simulink model "test6_1"  (R2014a)
settings: Solver=ode45  StartTime=0.0  StopTime=10.0  RelTol=1e-3
libraries: commrandsrc2 x1, commnoisgen2 x1
settings Model: Creator=asus  LastModifiedBy=asus

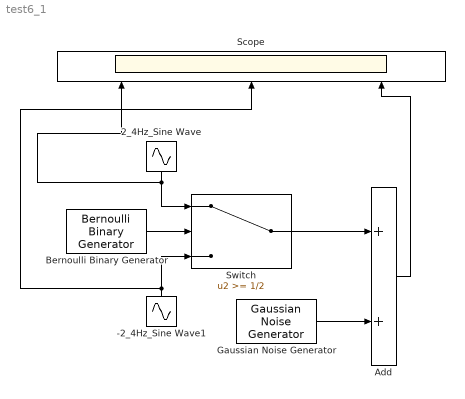
== system test6_1 ==
  -2_4Hz_Sine Wave1 : Sin  Amplitude=-2  Frequency=pi  SampleTime=1/8000
  2_4Hz_Sine Wave : Sin  Amplitude=2  Frequency=pi  SampleTime=1/8000
  Add : Sum
  Bernoulli Binary Generator : commrandsrc2/Bernoulli Binary Generator  P=1  seed=61  Ts=1  frameBased=off  sampPerFrame=1  orient=off  outDataType=double
  Gaussian Noise Generator : commnoisgen2/Gaussian Noise Generator  m=0  d=1  s=41  Ts=1  frameBased=off  sampPerFrame=1  orient=off  outDataType=double
  Scope : Scope  NumInputPorts=3
      settings: TimeRange=0.6999999999999993  YMin=-500~-2~-4  YMax=500~2~0
  Switch : Switch  Threshold=1/2
  wires:
  Bernoulli Binary Generator/1 -> Switch/2
  2_4Hz_Sine Wave/1 -> Scope/1, Switch/1
  -2_4Hz_Sine Wave1/1 -> Scope/2, Switch/3
  Gaussian Noise Generator/1 -> Add/2
  Switch/1 -> Add/1
  Add/1 -> Scope/3
